simulink model "rm_step_1"  (Simulink 8.7)
settings: Solver=VariableStepAuto  StartTime=0.0  StopTime=10  RelTol=1e-3
settings Model: Creator=admin  LastModifiedBy=admin
settings DataIOCC: LimitDataPoints=off  SaveFormat=Dataset
settings DebuggingCC: UnderspecifiedInitializationDetection=Simplified  MergeDetectMultiDrivingBlocksExec=error
settings HardwareCC: ProdBitPerPointer=64  ProdLargestAtomicFloat=Float  ProdIntDivRoundTo=Zero  ProdEndianess=LittleEndian  ProdWordSize=64  ProdHWDeviceType=Intel->x86-64 (Windows64)
settings ModelReferenceCC: PropagateSignalLabelsOutOfModel=on
settings ConfigComp: CovModelRefEnable=off

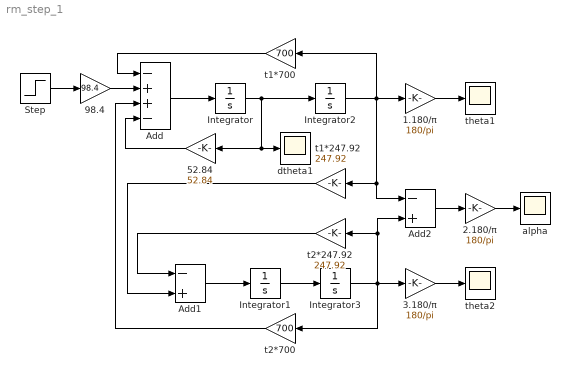
== system rm_step_1 ==
  " Integrator" : Integrator
  1.180/π : Gain  Gain=180/pi
  2.180/π : Gain  Gain=180/pi
  3.180/π : Gain  Gain=180/pi
  52.84 : Gain  Gain=52.84
  98.4 : Gain  Gain=98.4
  Add : Sum  Inputs=-++-
  Add1 : Sum  Inputs=-+
  Add2 : Sum  Inputs=-+
  Integrator1 : Integrator
  Integrator2 : Integrator
  Integrator3 : Integrator
  Step : Step  Time=0.01  SampleTime=0.005
  alpha : Scope
  dtheta1 : Scope
  t1*247.92 : Gain  Gain=247.92
  t1*700 : Gain  Gain=700
  t2*247.92 : Gain  Gain=247.92
  t2*700 : Gain  Gain=700
  theta1 : Scope
  theta2 : Scope
  wires:
  " Integrator"/1 -> Integrator2/1, dtheta1/1, 52.84/1
  Integrator1/1 -> Integrator3/1
  Integrator2/1 -> 1.180/π/1, Add2/1, t1*247.92/1, t1*700/1
  Add/1 -> " Integrator"/1
  52.84/1 -> Add/4
  t2*700/1 -> Add/3
  t1*700/1 -> Add/1
  98.4/1 -> Add/2
  t2*247.92/1 -> Add1/1
  Integrator3/1 -> 3.180/π/1, t2*700/1, Add2/2, t2*247.92/1
  Add1/1 -> Integrator1/1
  t1*247.92/1 -> Add1/2
  Step/1 -> 98.4/1
  1.180/π/1 -> theta1/1
  3.180/π/1 -> theta2/1
  2.180/π/1 -> alpha/1
  Add2/1 -> 2.180/π/1
